simulink library "calcSqredExpCov_ul"  (R2018b)
settings: Solver=VariableStepAuto  StartTime=0.0  StopTime=10.0  RelTol=1e-3
settings Model: Creator=asiddiq2  LastModifiedBy=asiddiq2

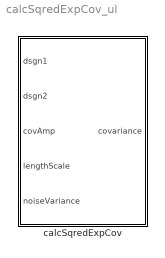
== system calcSqredExpCov_ul ==
  calcSqredExpCov : Subsystem

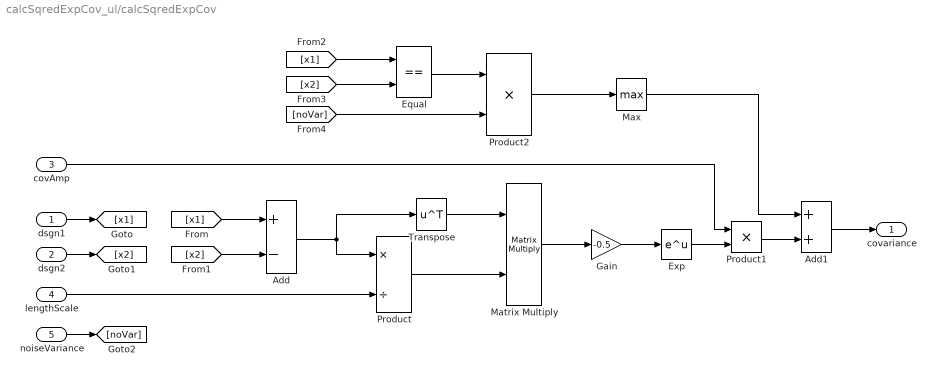
== system calcSqredExpCov_ul/calcSqredExpCov ==
  dsgn1 : Inport
  dsgn2 : Inport  Port=2
  covAmp : Inport  Port=3
  lengthScale : Inport  Port=4
  noiseVariance : Inport  Port=5
  Add : Sum  Inputs=+-
  Add1 : Sum
  Equal : RelationalOperator  Operator===  OutDataTypeStr=boolean  RndMeth=Simplest
  Exp : Math  SaturateOnIntegerOverflow=on
  Gain : Gain  Gain=-0.5
  Matrix Multiply : Product  Multiplication=Matrix(*)
  Max : MinMax  Function=max
  Product : Product  Inputs=*/
  Product1 : Product
  Product2 : Product
  Transpose : Math  Operator=transpose  SaturateOnIntegerOverflow=on
  covariance : Outport
  wires:
  dsgn1/1 -> [x1]
  dsgn2/1 -> [x2]
  Add/1 -> Transpose/1, Product/1
  lengthScale/1 -> Product/2
  Product/1 -> Matrix Multiply/2
  Transpose/1 -> Matrix Multiply/1
  Matrix Multiply/1 -> Gain/1
  Gain/1 -> Exp/1
  Exp/1 -> Product1/2
  Product1/1 -> Add1/2
  covAmp/1 -> Product1/1
  [x1] -> Add/1
  [x2] -> Add/2
  [x1] -> Equal/1
  [x2] -> Equal/2
  noiseVariance/1 -> [noVar]
  Add1/1 -> covariance/1
  Equal/1 -> Product2/1
  [noVar] -> Product2/2
  Product2/1 -> Max/1
  Max/1 -> Add1/1
